simulink model "DVA_sample"  (R2020b)
settings: Solver=VariableStepAuto  StartTime=0.0  StopTime=20  RelTol=1e-3
model workspace (MAT data in the model file):
  e = 0.05
  k1 = 55666
  k2 = 21012
  m = 0.244
  m1 = 44
  m2 = 5.5
  w = 47.499
libraries: simulink x2
settings Model: Creator=lenovo  LastModifiedBy=lenovo
settings SolverCC: ZeroCrossAlgorithm=Adaptive

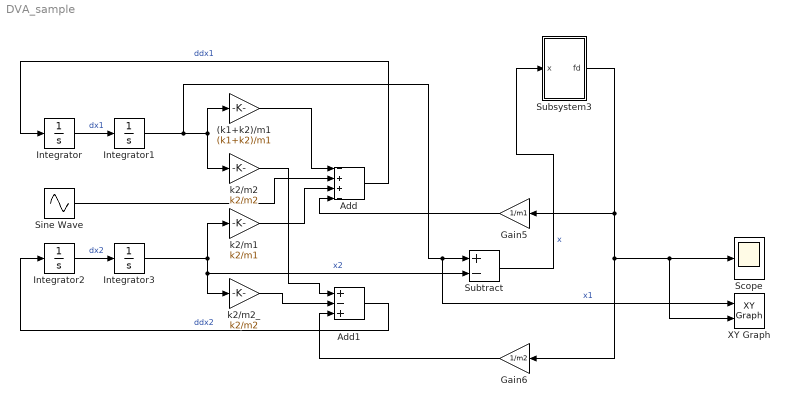
== system DVA_sample ==
  (k1+k2)/m1 : Gain  Gain=(k1+k2)/m1
  Add : Sum  Inputs=-++-
  Add1 : Sum  Inputs=+-+
  Gain5 : Gain  Gain=1/m1
  Gain6 : Gain  Gain=1/m2
  Integrator{,1..3} (4 alike) : Integrator
  Scope : Scope
  Sine Wave : Sin  Amplitude=(m*e*w^2)/m1  Frequency=w  SampleTime=0
  Subsystem3 : Subsystem
  Subtract : Sum  Inputs=+-
  XY Graph : simulink/Sinks/XY Graph  xmin=0  xmax=0.001  ymin=-40  ymax=40  st=-1
  k2/m1 : Gain  Gain=k2/m1
  k2/m2 : Gain  Gain=k2/m2
  k2/m2_ : Gain  Gain=k2/m2
  wires:
  Integrator/1 -> Integrator1/1  "dx1"
  Integrator1/1 -> XY Graph/1, Subtract/1, k2/m2/1, (k1+k2)/m1/1  "x1"
  Integrator2/1 -> Integrator3/1  "dx2"
  Integrator3/1 -> Subtract/2, k2/m2_/1, k2/m1/1  "x2"
  Sine Wave/1 -> Add/2
  k2/m1/1 -> Add/3
  (k1+k2)/m1/1 -> Add/1
  Add/1 -> Integrator/1  "ddx1"
  k2/m2_/1 -> Add1/2
  k2/m2/1 -> Add1/1
  Add1/1 -> Integrator2/1  "ddx2"
  Subtract/1 -> Subsystem3/1(x)  "x"
  Gain5/1 -> Add/4
  Gain6/1 -> Add1/3
  Subsystem3/1(fd) -> Gain6/1, XY Graph/2, Scope/1, Gain5/1

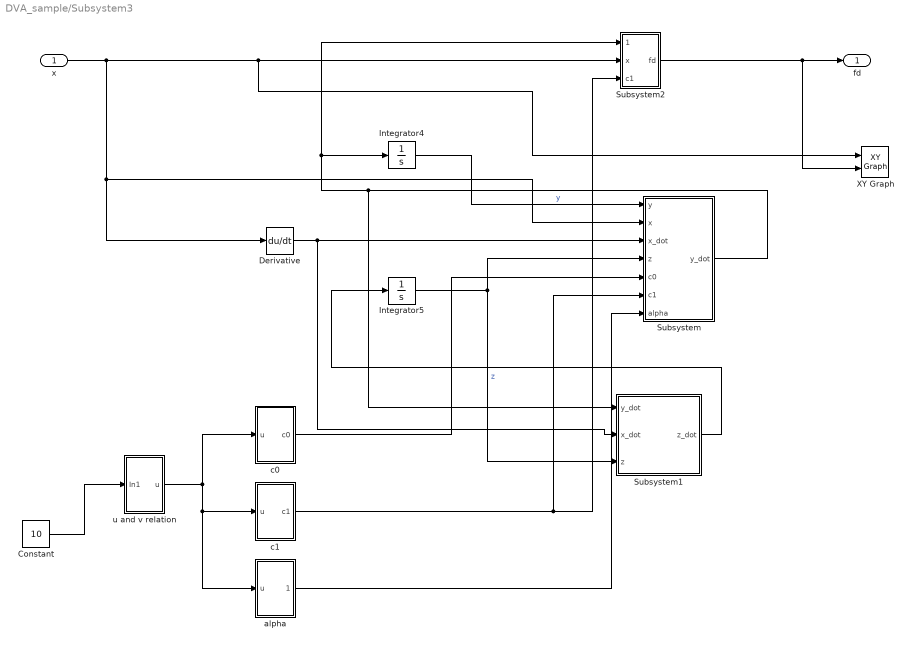
== system DVA_sample/Subsystem3 ==
  x : Inport
  Constant : Constant  Value=10
  Derivative : Derivative
  Integrator4 : Integrator
  Integrator5 : Integrator
  Subsystem : Subsystem
  Subsystem1 : Subsystem
  Subsystem2 : Subsystem
  XY Graph : simulink/Sinks/XY Graph  xmin=-.5  xmax=.5  ymin=-5000  ymax=5000  st=-1
  alpha : Subsystem
  c0 : Subsystem
  c1 : Subsystem
  u and v relation : Subsystem
  fd : Outport
  wires:
  Constant/1 -> u and v relation/1(In1)
  Subsystem/1(y_dot) -> Subsystem1/1(y_dot), Integrator4/1, Subsystem2/1(y_dot)
  Integrator5/1 -> Subsystem1/3(z), Subsystem/4(z)  "z"
  c0/1(c0) -> Subsystem/5(c0)
  u and v relation/1(u) -> alpha/1(u), c1/1(u), c0/1(u)
  x/1 -> Derivative/1, Subsystem/2(x), XY Graph/1, Subsystem2/2(x)
  c1/1(c1) -> Subsystem2/3(c1), Subsystem/6(c1)
  Subsystem1/1(z_dot) -> Integrator5/1
  Integrator4/1 -> Subsystem/1(y)  "y"
  Derivative/1 -> Subsystem1/2(x_dot), Subsystem/3(x_dot)
  alpha/1(alpha) -> Subsystem/7(alpha)
  Subsystem2/1(fd) -> XY Graph/2, fd/1

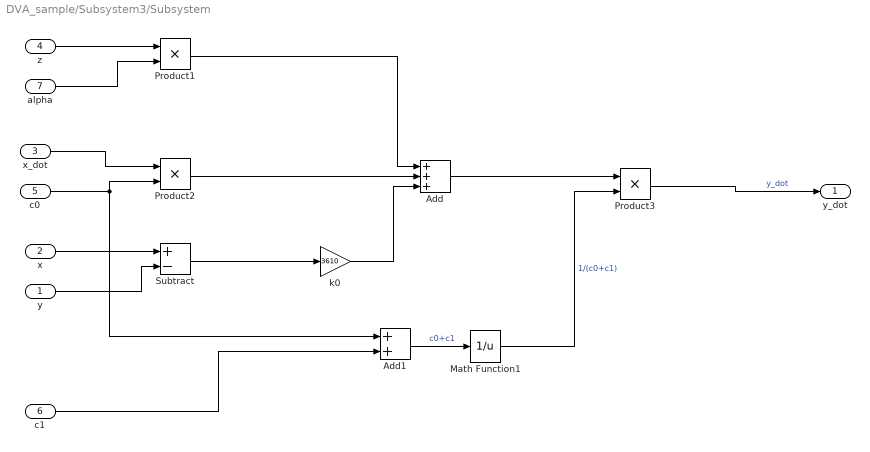
== system DVA_sample/Subsystem3/Subsystem ==
  y : Inport
  x : Inport  Port=2
  x_dot : Inport  Port=3
  z : Inport  Port=4
  c0 : Inport  Port=5
  c1 : Inport  Port=6
  alpha : Inport  Port=7
  Add : Sum  Inputs=+++
  Add1 : Sum
  Math Function1 : Math  Operator=reciprocal  SaturateOnIntegerOverflow=on
  Product1 : Product
  Product2 : Product
  Product3 : Product
  Subtract : Sum  Inputs=+-
  k0 : Gain  Gain=3610
  y_dot : Outport
  wires:
  Product1/1 -> Add/1
  Subtract/1 -> k0/1
  Add1/1 -> Math Function1/1  "c0+c1"
  k0/1 -> Add/3
  Math Function1/1 -> Product3/2  "1/(c0+c1)"
  c0/1 -> Add1/1, Product2/2
  z/1 -> Product1/1
  Product3/1 -> y_dot/1  "y_dot"
  Add/1 -> Product3/1
  Product2/1 -> Add/2
  y/1 -> Subtract/2
  x/1 -> Subtract/1
  c1/1 -> Add1/2
  x_dot/1 -> Product2/1
  alpha/1 -> Product1/2

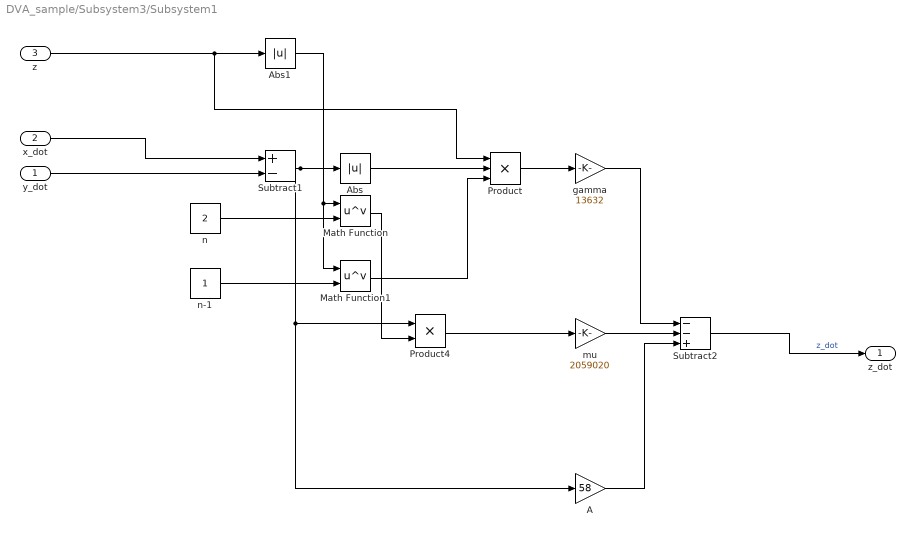
== system DVA_sample/Subsystem3/Subsystem1 ==
  y_dot : Inport
  x_dot : Inport  Port=2
  z : Inport  Port=3
  A : Gain  Gain=58
  Abs : Abs
  Abs1 : Abs
  Math Function : Math  Operator=pow  SaturateOnIntegerOverflow=on
  Math Function1 : Math  Operator=pow  SaturateOnIntegerOverflow=on
  Product : Product  Inputs=3
  Product4 : Product
  Subtract1 : Sum  Inputs=+-
  Subtract2 : Sum  Inputs=--+
  gamma : Gain  Gain=13632
  mu : Gain  Gain=2059020
  n : Constant  Value=2
  n-1 : Constant
  z_dot : Outport
  wires:
  Abs/1 -> Product/2
  Subtract1/1 -> A/1, Product4/1, Abs/1
  n/1 -> Math Function/2
  Abs1/1 -> Math Function1/1, Math Function/1
  gamma/1 -> Subtract2/1
  z/1 -> Abs1/1, Product/1
  mu/1 -> Subtract2/2
  Product4/1 -> mu/1
  Math Function/1 -> Product4/2
  Math Function1/1 -> Product/3
  Product/1 -> gamma/1
  y_dot/1 -> Subtract1/2
  Subtract2/1 -> z_dot/1  "z_dot"
  x_dot/1 -> Subtract1/1
  A/1 -> Subtract2/3
  n-1/1 -> Math Function1/2

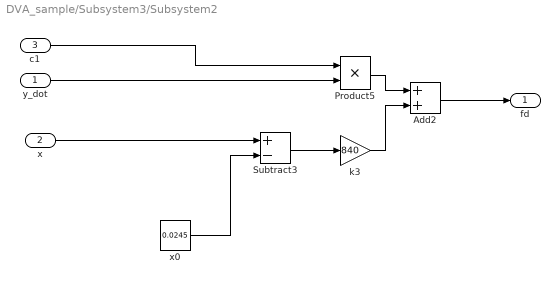
== system DVA_sample/Subsystem3/Subsystem2 ==
  y_dot : Inport
  x : Inport  Port=2
  c1 : Inport  Port=3
  Add2 : Sum
  Product5 : Product
  Subtract3 : Sum  Inputs=+-
  k3 : Gain  Gain=840
  x0 : Constant  Value=0.0245
  fd : Outport
  wires:
  Subtract3/1 -> k3/1
  y_dot/1 -> Product5/2
  Product5/1 -> Add2/1
  k3/1 -> Add2/2
  Add2/1 -> fd/1
  x0/1 -> Subtract3/2
  c1/1 -> Product5/1
  x/1 -> Subtract3/1

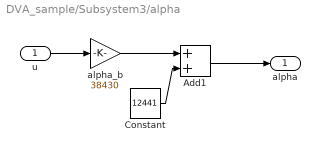
== system DVA_sample/Subsystem3/alpha ==
  u : Inport
  Add1 : Sum
  Constant : Constant  Value=12441
  alpha_b : Gain  Gain=38430
  alpha : Outport
  wires:
  Add1/1 -> alpha/1
  Constant/1 -> Add1/2
  alpha_b/1 -> Add1/1
  u/1 -> alpha_b/1

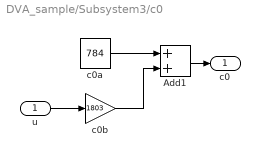
== system DVA_sample/Subsystem3/c0 ==
  u : Inport
  Add1 : Sum
  c0a : Constant  Value=784
  c0b : Gain  Gain=1803
  c0 : Outport
  wires:
  c0b/1 -> Add1/2
  c0a/1 -> Add1/1
  u/1 -> c0b/1
  Add1/1 -> c0/1

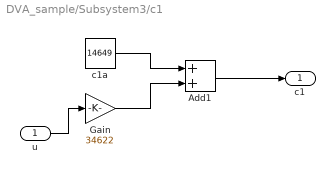
== system DVA_sample/Subsystem3/c1 ==
  u : Inport
  " c1a" : Constant  Value=14649
  Add1 : Sum
  Gain : Gain  Gain=34622
  c1 : Outport
  wires:
  Gain/1 -> Add1/2
  " c1a"/1 -> Add1/1
  Add1/1 -> c1/1
  u/1 -> Gain/1

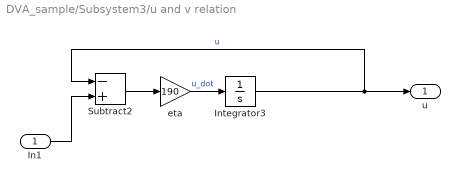
== system DVA_sample/Subsystem3/u and v relation ==
  In1 : Inport
  Integrator3 : Integrator
  Subtract2 : Sum  Inputs=-+
  eta : Gain  Gain=190
  u : Outport
  wires:
  Subtract2/1 -> eta/1
  In1/1 -> Subtract2/2
  Integrator3/1 -> u/1, Subtract2/1  "u"
  eta/1 -> Integrator3/1  "u_dot"
